simulink model "sys_nl"  (R2023b)
settings: Solver=VariableStepAuto  StartTime=0.0  StopTime=30  RelTol=1e-3
values from neighbouring files (symbols this model uses):
  u_nom = 0    [system_configuration.m]
  y_nom = [0 0]    [system_configuration.m]
settings Model: Creator=aniello  LastModifiedBy=aniello

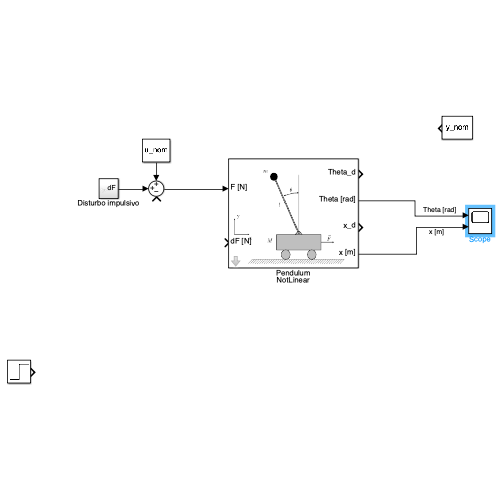
[thumbnail: Simulink's stored preview of the top-level diagram]
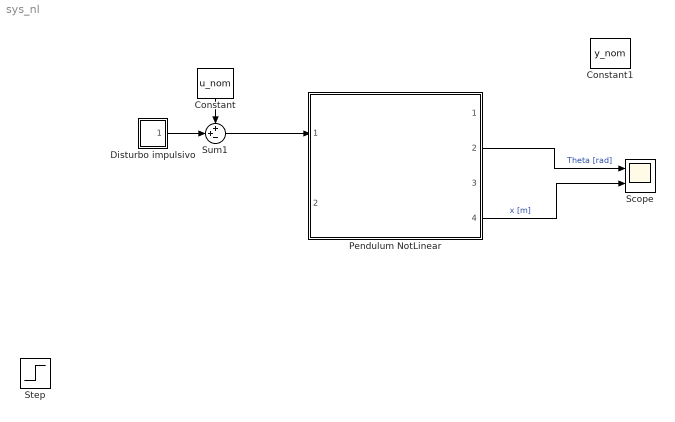
== system sys_nl ==
  Constant : Constant  Value=u_nom
  Constant1 : Constant  Value=y_nom
  Disturbo impulsivo : Subsystem
  Pendulum NotLinear : Subsystem  ReferencedSubsystem=pendulum
  Scope : Scope  NumInputPorts=2
  Step : Step  SampleTime=0
  Sum1 : Sum  Inputs=++-
  wires:
  Sum1/1 -> Pendulum NotLinear/1
  Pendulum NotLinear/2 -> Scope/1  "Theta [rad]"
  Constant/1 -> Sum1/1
  Pendulum NotLinear/4 -> Scope/2  "x [m]"
  Disturbo impulsivo/1(dF) -> Sum1/2

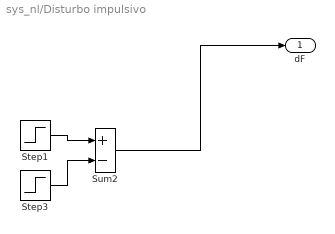
== system sys_nl/Disturbo impulsivo ==
  Step1 : Step  Time=0  After=2  SampleTime=0
  Step3 : Step  Time=0.5  SampleTime=0
  Sum2 : Sum  Inputs=+-
  dF : Outport
  wires:
  Sum2/1 -> dF/1
  Step3/1 -> Sum2/2
  Step1/1 -> Sum2/1
